simulink model "Uncompensated_Model"  (R2019b)
settings: Solver=VariableStepAuto  StartTime=0.0  StopTime=10.0  RelTol=1e-3
settings Model: Creator=EASY LIFE  LastModifiedBy=EASY LIFE

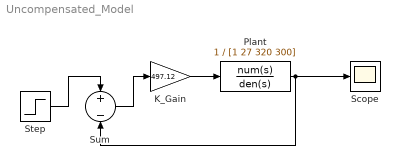
== system Uncompensated_Model ==
  K_Gain : Gain  Gain=497.12
  Plant : TransferFcn  Numerator=1  Denominator=[1 27 320 300]
  Scope : Scope
  Step : Step  SampleTime=0
  Sum : Sum  Inputs=+-
  wires:
  Step/1 -> Sum/1
  Sum/1 -> K_Gain/1
  K_Gain/1 -> Plant/1
  Plant/1 -> Scope/1, Sum/2
